simulink model "GFLI_L"  (R2024b)
settings: Solver=ode4  StartTime=0.0  StopTime=13  FixedStep=Tsam  RelTol=1e-3
values from neighbouring files (symbols this model uses):
  I2d = 3195    [GFLI_meas.m]    (also in SameOP_DifferParams.m; SameOP_Params_DifferConfig.m)
  I2q = -2132    [GFLI_meas.m]    (also in SameOP_DifferParams.m = 0; SameOP_Params_DifferConfig.m = 0)
  Kii = 0.0348    [GFLI_meas.m]
  Kipll = 400/(Vdc/2)    (= 0.695652173913)    [GFLI_meas.m]
  Kpi = 1.7391e-4    (= 0.00017391)    [GFLI_meas.m]
  Kppll = 40/(Vdc/2)    (= 0.0695652173913)    [GFLI_meas.m]
  Lf1 = 250e-6    (= 0.00025)    [GFLI_meas.m]
  Rf1 = 3e-3    (= 0.003)    [GFLI_meas.m]
  s = tf('s')    [GFLI_meas.m]    (also in GFLI_meas_PlotYddYqq.m; SameOP_DifferParams.m)
  Td = 1.5*Ts    (= 0.0003)    [GFLI_meas.m]    (also in GFLI_meas_PlotYddYqq.m = p.Td; SameOP_DifferParams.m = p.Td)
  Tsam = 5e-5    (= 5e-05)    [GFLI_meas.m]
  Vdc = 1150    [GFLI_meas.m]
  Vg = 575    [GFLI_meas.m]
  w = w_meas    [GFLI_meas.m]
  w1 = 2*pi*f0    (= 314.159265359)    [GFLI_meas.m]    (also in GFLI_meas_PlotYddYqq.m)
  w_meas = 2*pi*fHz_meas    [GFLI_meas.m]    (also in GFLI_meas_PlotYddYqq.m; SameOP_DifferParams.m; SameOP_Params_DifferConfig.m)
undefined symbols (not defined in the file or in its folder): DiscIntNeverNeededParam
libraries: slctrl_fre x12, spsControlledVoltageSourceLib x6, spsabctodq0Lib x5, slctrl_signal x4, spsACVoltageSourceLib x3, spsSeriesRLCBranchLib x3, spsdq0toabcLib x2, spsThreePhaseVIMeasurementLib x2, spsPLL3phLib x1, spsGroundLib x1, sps_lib x1
(part 1 of 2)
settings Model: SimulationMode=accelerator  Creator=ACER  LastModifiedBy=ACER
settings DataIOCC: SaveFormat=StructureWithTime  SignalLogging=off  DSMLogging=off  SaveTime=off  ReturnWorkspaceOutputs=off

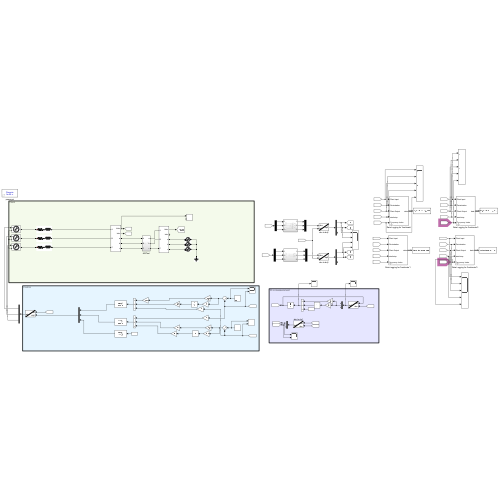
[thumbnail: Simulink's stored preview of the top-level diagram]
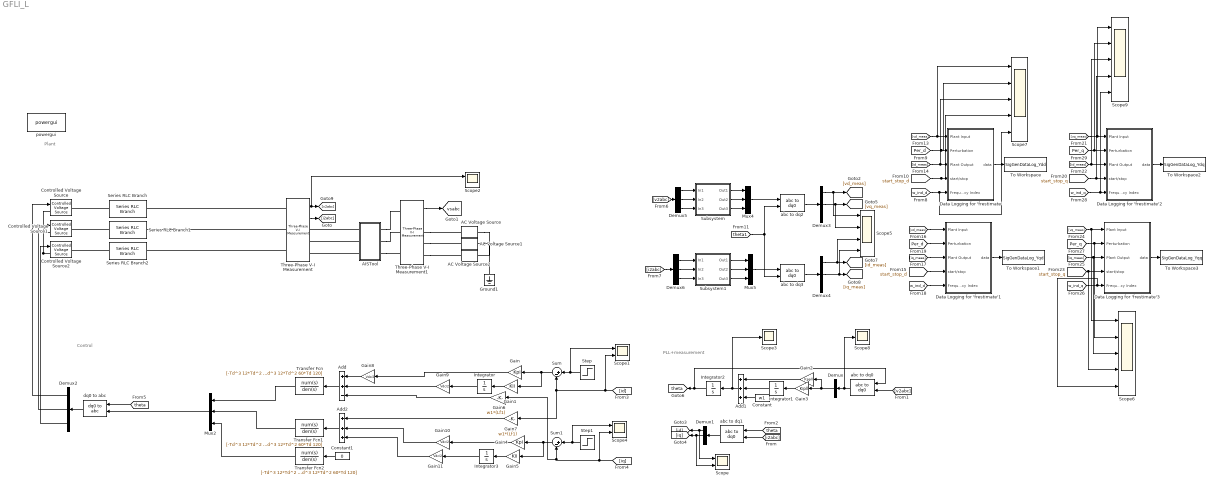
== system GFLI_L ==
  note: Plant
  note: Control
  note: PLL+measurement
  AC Voltage Source : spsACVoltageSourceLib/AC Voltage Source  Amplitude=Vg  Phase=0  Frequency=50  SampleTime=0  Measurements=None  BusType=swing  Pref=10e3  Qref=0  Qmin=-inf  Qmax=+inf
  AC Voltage Source1 : spsACVoltageSourceLib/AC Voltage Source  Amplitude=Vg  Phase=-120  Frequency=50  SampleTime=0  Measurements=None  BusType=swing  Pref=10e3  Qref=0  Qmin=-inf  Qmax=+inf
  AC Voltage Source2 : spsACVoltageSourceLib/AC Voltage Source  Amplitude=Vg  Phase=120  Frequency=50  SampleTime=0  Measurements=None  BusType=swing  Pref=10e3  Qref=0  Qmin=-inf  Qmax=+inf
  AISTool : Subsystem
  Add : Sum  Inputs=++-
  Add1 : Sum  Inputs=+++
  Add2 : Sum  Inputs=+++
  Constant : Constant  Value=w1
  Constant1 : Constant  Value=0
  Controlled Voltage Source : spsControlledVoltageSourceLib/Controlled Voltage Source  Initialize=on  Source_Type=AC  Amplitude=0  Phase=0  Frequency=0  Measurements=None
  Controlled Voltage Source1 : spsControlledVoltageSourceLib/Controlled Voltage Source  Initialize=on  Source_Type=AC  Amplitude=0  Phase=0  Frequency=0  Measurements=None
  Controlled Voltage Source2 : spsControlledVoltageSourceLib/Controlled Voltage Source  Initialize=on  Source_Type=AC  Amplitude=0  Phase=0  Frequency=0  Measurements=None
  Data Logging for 'frestimate' : Subsystem  mask(Companion Data Logger){Ts=Tsam, SignalType=Sinestream, FrequenciesSS=w_meas, FreqUnitsSS=rad/s, NumOfSetPeriod=1, NumOfEstPeriod=2, PRBSNumOfPeriod=1, FrequenciesSI=w, FreqUnitsSI=rad/s, NumOfPeriodLowestFreq=3, ReadySignalActiveChoice=VariantSinestream, InfoSignalActiveChoice=VariantSinestream}
      mask prompts: Ts "Sample Time (Ts)"; SignalType "Input Signal Type"; FrequenciesSS "Frequencies Vector"; NumOfSetPeriod "Number of Settling Periods"; NumOfEstPeriod "Number of Estimation Periods"; PRBSNumOfPeriod "Number of PRBS Signal Periods"; FrequenciesSI "Frequencies Vector"; NumOfPeriodLowestFreq "Number of  periods of the lowest frequency"; ReadySignalActiveChoice "Simulink:Variants:LabelComboBox"; InfoSignalActiveChoice "Simulink:Variants:LabelComboBox"
      mask help: Log data from signal generator blocks to work with "frestimate" API or frequency response estimation.
      mask init:
      | IsSinestreamSignal = strcmpi(get_param(gcb,'SignalType'),'Sinestream');
      |     IsSuperpositionSignal = strcmpi(get_param(gcb,'SignalType'),'Superposition');
      |     IsPRBSSignal = strcmpi(get_param(gcb,'SignalType'),'PRBS');
      |     IsHz = false;
      |     maskObj = Simulink.Mask.get(gcb);
      |     objectSinestream = maskObj.getDialogControl('SinestreamPanel');
      |     objectSuperposition = maskObj.getDialogControl('SuperpositionPanel');
      |     objectPRBS = maskObj.getDialogControl('PRBSPanel');
      |     %% Update optional inports
      |     inport_name = {'Frequency Index'};
      |     AvailableBlocks = get_param(gcb,'Blocks');
      |     % what exists in the block (old)
      |     type_in_block = ismember(inport_name,AvailableBlocks);
      |     % what is specified in the dialog (new)
      |     type_in_mask = IsSinestreamSignal;
      |     if IsSinestreamSignal
      |         objectSinestream.Visible = 'on';
      |         objectSuperposition.Visible = 'off';
      |         objectPRBS.Visible = 'off';
      |         set_param(gcb,'ReadySignalActiveChoice','VariantSinestream');  
      |         set_param(gcb,'InfoSignalActiveChoice','VariantSinestream');        
      |         IsHz = strcmpi(get_param(gcb,'FreqUnitsSS'),'Hz');
      |     elseif IsPRBSSignal
      |         objectSinestream.Visible = 'off';
      |         objectSuperposition.Visible = 'off';
      |         objectPRBS.Visible = 'on';
      |         set_param(gcb,'ReadySignalActiveChoice','VariantPRBS');  
      |         set_param(gcb,'InfoSignalActiveChoice','VariantPRBS');    
      |     else
      |         objectSinestream.Visible = 'off';
      |         objectSuperposition.Visible = 'on';
      |         objectPRBS.Visible = 'off';
      |         set_param(gcb,'ReadySignalActiveChoice','VariantSuperposition');  
      |         set_param(gcb,'InfoSignalActiveChoice','VariantSuperposition');    
      |         IsHz = strcmpi(get_param(gcb,'FreqUnitsSI'),'Hz');
      |     end
      |     % Update Inport
      |     port = 5;
      |     port = slctrlblkdlgs.OnlinePIDTuner.utilUpdateInport(gcb,'RateTransition_idx',AvailableBlocks,type_in_mask,type_in_block,1,'Frequency Index',port,1,'FrequenciesSS','double');
      |     if IsHz
      |         ConvFactor = 2*pi;
      |     else
      |         ConvFactor = 1;
      |     end
      mask Help: eval(open("block_data_logging_for_frestimate.html"));
      mask TypeOptions SignalType: Sinestream | Superposition | PRBS
      mask TypeOptions FreqUnitsSS: rad/s | Hz
      mask TypeOptions FreqUnitsSI: rad/s | Hz
      mask TypeOptions ReadySignalActiveChoice: Generate Ready Signal/LabelModeActiveChoice
      mask TypeOptions InfoSignalActiveChoice: Generate Info Signal/LabelModeActiveChoice
      mask DialogControl Container3 Prompt: Signal Specific Settings
      mask DialogControl ReadySignalActiveChoice Prompt: Label mode active choice:
      mask DialogControl InfoSignalActiveChoice Prompt: Label mode active choice:
  Data Logging for 'frestimate'1 : Subsystem  mask(Companion Data Logger){Ts=Tsam, SignalType=Sinestream, FrequenciesSS=w_meas, FreqUnitsSS=rad/s, NumOfSetPeriod=1, NumOfEstPeriod=2, PRBSNumOfPeriod=1, FrequenciesSI=w, FreqUnitsSI=rad/s, NumOfPeriodLowestFreq=3, ReadySignalActiveChoice=VariantSinestream, InfoSignalActiveChoice=VariantSinestream}
      mask prompts: Ts "Sample Time (Ts)"; SignalType "Input Signal Type"; FrequenciesSS "Frequencies Vector"; NumOfSetPeriod "Number of Settling Periods"; NumOfEstPeriod "Number of Estimation Periods"; PRBSNumOfPeriod "Number of PRBS Signal Periods"; FrequenciesSI "Frequencies Vector"; NumOfPeriodLowestFreq "Number of  periods of the lowest frequency"; ReadySignalActiveChoice "Simulink:Variants:LabelComboBox"; InfoSignalActiveChoice "Simulink:Variants:LabelComboBox"
      mask help: Log data from signal generator blocks to work with "frestimate" API or frequency response estimation.
      mask init: same as GFLI_L/Data Logging for 'frestimate'
      mask Help: eval(open("block_data_logging_for_frestimate.html"));
      mask TypeOptions SignalType: Sinestream | Superposition | PRBS
      mask TypeOptions FreqUnitsSS: rad/s | Hz
      mask TypeOptions FreqUnitsSI: rad/s | Hz
      mask TypeOptions ReadySignalActiveChoice: Generate Ready Signal/LabelModeActiveChoice
      mask TypeOptions InfoSignalActiveChoice: Generate Info Signal/LabelModeActiveChoice
      mask DialogControl Container3 Prompt: Signal Specific Settings
      mask DialogControl ReadySignalActiveChoice Prompt: Label mode active choice:
      mask DialogControl InfoSignalActiveChoice Prompt: Label mode active choice:
  Data Logging for 'frestimate'2 : Subsystem  mask(Companion Data Logger){Ts=Tsam, SignalType=Sinestream, FrequenciesSS=w_meas, FreqUnitsSS=rad/s, NumOfSetPeriod=1, NumOfEstPeriod=2, PRBSNumOfPeriod=1, FrequenciesSI=w, FreqUnitsSI=rad/s, NumOfPeriodLowestFreq=3, ReadySignalActiveChoice=VariantSinestream, InfoSignalActiveChoice=VariantSinestream}
      mask prompts: Ts "Sample Time (Ts)"; SignalType "Input Signal Type"; FrequenciesSS "Frequencies Vector"; NumOfSetPeriod "Number of Settling Periods"; NumOfEstPeriod "Number of Estimation Periods"; PRBSNumOfPeriod "Number of PRBS Signal Periods"; FrequenciesSI "Frequencies Vector"; NumOfPeriodLowestFreq "Number of  periods of the lowest frequency"; ReadySignalActiveChoice "Simulink:Variants:LabelComboBox"; InfoSignalActiveChoice "Simulink:Variants:LabelComboBox"
      mask help: Log data from signal generator blocks to work with "frestimate" API or frequency response estimation.
      mask init: same as GFLI_L/Data Logging for 'frestimate'
      mask Help: eval(open("block_data_logging_for_frestimate.html"));
      mask TypeOptions SignalType: Sinestream | Superposition | PRBS
      mask TypeOptions FreqUnitsSS: rad/s | Hz
      mask TypeOptions FreqUnitsSI: rad/s | Hz
      mask TypeOptions ReadySignalActiveChoice: Generate Ready Signal/LabelModeActiveChoice
      mask TypeOptions InfoSignalActiveChoice: Generate Info Signal/LabelModeActiveChoice
      mask DialogControl Container3 Prompt: Signal Specific Settings
      mask DialogControl ReadySignalActiveChoice Prompt: Label mode active choice:
      mask DialogControl InfoSignalActiveChoice Prompt: Label mode active choice:
  Data Logging for 'frestimate'3 : Subsystem  mask(Companion Data Logger){Ts=Tsam, SignalType=Sinestream, FrequenciesSS=w_meas, FreqUnitsSS=rad/s, NumOfSetPeriod=1, NumOfEstPeriod=2, PRBSNumOfPeriod=1, FrequenciesSI=w, FreqUnitsSI=rad/s, NumOfPeriodLowestFreq=3, ReadySignalActiveChoice=VariantSinestream, InfoSignalActiveChoice=VariantSinestream}
      mask prompts: Ts "Sample Time (Ts)"; SignalType "Input Signal Type"; FrequenciesSS "Frequencies Vector"; NumOfSetPeriod "Number of Settling Periods"; NumOfEstPeriod "Number of Estimation Periods"; PRBSNumOfPeriod "Number of PRBS Signal Periods"; FrequenciesSI "Frequencies Vector"; NumOfPeriodLowestFreq "Number of  periods of the lowest frequency"; ReadySignalActiveChoice "Simulink:Variants:LabelComboBox"; InfoSignalActiveChoice "Simulink:Variants:LabelComboBox"
      mask help: Log data from signal generator blocks to work with "frestimate" API or frequency response estimation.
      mask init: same as GFLI_L/Data Logging for 'frestimate'
      mask Help: eval(open("block_data_logging_for_frestimate.html"));
      mask TypeOptions SignalType: Sinestream | Superposition | PRBS
      mask TypeOptions FreqUnitsSS: rad/s | Hz
      mask TypeOptions FreqUnitsSI: rad/s | Hz
      mask TypeOptions ReadySignalActiveChoice: Generate Ready Signal/LabelModeActiveChoice
      mask TypeOptions InfoSignalActiveChoice: Generate Info Signal/LabelModeActiveChoice
      mask DialogControl Container3 Prompt: Signal Specific Settings
      mask DialogControl ReadySignalActiveChoice Prompt: Label mode active choice:
      mask DialogControl InfoSignalActiveChoice Prompt: Label mode active choice:
  Demux{,1..6} (7 alike) : Demux  Outputs=3
  Gain : Gain  Gain=Kpi
  Gain1 : Gain  Gain=Kii
  Gain{8..11} (4 alike) : Gain  Gain=Vdc/2
  Gain2 : Gain  Gain=Kppll
  Gain3 : Gain  Gain=Kipll
  Gain4 : Gain  Gain=Kpi
  Gain5 : Gain  Gain=Kii
  Gain6 : Gain  Gain=w1*(Lf1)
  Gain7 : Gain  Gain=w1*(Lf1)
  Ground1 : spsGroundLib/Ground  LConnTagsString=a
  Integrator{,1..3} (4 alike) : Integrator
  Mux2 : Mux  Inputs=3
  Mux4 : Mux  Inputs=3
  Mux5 : Mux  Inputs=3
  Scope{,1..2,4} (4 alike) : Scope  NumInputPorts=2
  Scope3 : Scope
  Scope5 : Scope  NumInputPorts=4
  Scope6 : Scope  NumInputPorts=5
  Scope7 : Scope  NumInputPorts=5
  Scope8 : Scope
  Scope9 : Scope  NumInputPorts=5
  Series RLC Branch : spsSeriesRLCBranchLib/Series RLC Branch  LConnTagsString=__new0  RConnTagsString=__new0  BranchType=RL  Resistance=Rf1  Inductance=Lf1  SetiL0=off  InitialCurrent=0  Capacitance=1e-6  Setx0=off  InitialVoltage=0  Measurements=None
  Series RLC Branch1 : spsSeriesRLCBranchLib/Series RLC Branch  LConnTagsString=__new0  RConnTagsString=__new0  BranchType=RL  Resistance=Rf1  Inductance=Lf1  SetiL0=off  InitialCurrent=0  Capacitance=1e-6  Setx0=off  InitialVoltage=0  Measurements=None
  Series RLC Branch2 : spsSeriesRLCBranchLib/Series RLC Branch  LConnTagsString=__new0  RConnTagsString=__new0  BranchType=RL  Resistance=Rf1  Inductance=Lf1  SetiL0=off  InitialCurrent=0  Capacitance=1e-6  Setx0=off  InitialVoltage=0  Measurements=None
  Step : Step  Time=2  Before=I2d  After=I2d  SampleTime=0
  Step1 : Step  Time=3  Before=I2q  After=I2q  SampleTime=0
  Subsystem : Subsystem
  Subsystem1 : Subsystem
  Sum : Sum  Inputs=|+-
  Sum1 : Sum  Inputs=|+-
  Three-Phase V-I Measurement : spsThreePhaseVIMeasurementLib/Three-Phase V-I Measurement  VoltageMeasurement=phase-to-ground  SetLabelV=off  LabelV=Vabc  Vpu=off  VpuLL=off  CurrentMeasurement=yes  SetLabelI=off  LabelI=Iabc  Ipu=off  Pbase=100e6  Vbase=500e3  OutputType=Complex  PhasorSimulation=off  PSBequivalent=0
  Three-Phase V-I Measurement1 : spsThreePhaseVIMeasurementLib/Three-Phase V-I Measurement  VoltageMeasurement=phase-to-ground  SetLabelV=off  LabelV=Vabc  Vpu=off  VpuLL=off  CurrentMeasurement=yes  SetLabelI=off  LabelI=Iabc  Ipu=off  Pbase=100e6  Vbase=500e3  OutputType=Complex  PhasorSimulation=off  PSBequivalent=0
  To Workspace : ToWorkspace  VariableName=SigGenDataLog_Ydd  SaveFormat=Timeseries  SampleTime=5e-5
  To Workspace1 : ToWorkspace  VariableName=SigGenDataLog_Yqd  SaveFormat=Timeseries  SampleTime=5e-5
  To Workspace2 : ToWorkspace  VariableName=SigGenDataLog_Ydq  SaveFormat=Timeseries  SampleTime=5e-5
  To Workspace3 : ToWorkspace  VariableName=SigGenDataLog_Yqq  SaveFormat=Timeseries  SampleTime=5e-5
  Transfer Fcn : TransferFcn  Numerator=[-Td^3 12*Td^2 -60*Td 120]  Denominator=[Td^3 12*Td^2 60*Td 120]
  Transfer Fcn1 : TransferFcn  Numerator=[-Td^3 12*Td^2 -60*Td 120]  Denominator=[Td^3 12*Td^2 60*Td 120]
  Transfer Fcn2 : TransferFcn  Numerator=[-Td^3 12*Td^2 -60*Td 120]  Denominator=[Td^3 12*Td^2 60*Td 120]
  abc to dq{0..3} (4 alike) : spsabctodq0Lib/abc to dq0  Alignment=Aligned with phase A axis
  dq0 to abc : spsdq0toabcLib/dq0 to abc  Alignment=Aligned with phase A axis
  powergui : sps_lib/powergui  Priority=1  SimulationMode=Discrete  SampleTime=Tsam  frequency=60  Iterations=50  frequencyindice=0  Pbase=100e6  ErrMax=1e-4  UnitsV=kV  UnitsW=MW  buscounter=0  FunctionMessages=off  echomessages=off  EnableUseOfTLC=off  CurrentSourceSwitches=off  DisableSnubberDevices=off  DisableRonSwitches=off  DisableVfSwitches=off  DisplayEquations=off  AutomaticDiscreteSolvers=off  SolverType=Tustin/Backward Euler (TBE)  Interpol=off  ExternalGateDelay=off  methode=off  Ts=100  x0status=zero  SPID=on  SwTol=0  HookPort=off  NonlinearTolerance=1e-4  nMaxIteration=100  ContinueOnMaxIteration=off  RestoreLinks=warning  ResistiveCurrentMeasurement=off  Frange=[0:2:500]  Ylog=off  Xlog=on  ShowGrid=off  save=off  variable=ZData  structure=0  ZoomFFT=off  StartTime=0.0  cycles=1  DisplayStyle=1  fundamental=60  FreqAxis=off  MaxFrequency=1000  frequencyindicesteady=1  RmsSteady=1  display=off
  tag scope: theta=global, vsabc=global
  wires:
  Demux1/2 -> Scope/2, [iq]
  Mux2/1 -> dq0 to abc/1
  Demux/2 -> Gain2/1, Gain3/1
  Demux2/3 -> Controlled Voltage Source2/1
  [theta] -> dq0 to abc/2
  Gain5/1 -> Integrator3/1
  Integrator2/1 -> [theta], abc to dq0/2
  dq0 to abc/1 -> Demux2/1
  Add2/1 -> Transfer Fcn1/1
  [theta] -> abc to dq1/2
  Demux2/2 -> Controlled Voltage Source1/1
  Gain/1 -> Gain8/1
  Add/1 -> Transfer Fcn/1
  Gain9/1 -> Add/2
  Integrator3/1 -> Gain11/1
  [iq] -> Scope4/2, Gain6/1, Sum1/2
  Add1/1 -> Scope3/1, Integrator2/1
  Transfer Fcn2/1 -> Mux2/3
  Gain1/1 -> Integrator/1
  Transfer Fcn/1 -> Mux2/1
  [i2abc] -> abc to dq1/1
  Sum1/1 -> Gain4/1, Gain5/1
  Gain8/1 -> Add/1
  Sum/1 -> Gain1/1, Gain/1
  Gain4/1 -> Gain10/1
  Gain11/1 -> Add2/3
  Constant/1 -> Add1/3
  Step1/1 -> Scope4/1, Sum1/1
  Integrator1/1 -> Add1/2
  Gain2/1 -> Add1/1
  Gain3/1 -> Integrator1/1
  abc to dq0/1 -> Scope8/1, Demux/1
  Transfer Fcn1/1 -> Mux2/2
  Demux1/1 -> Scope/1, [id]
  Constant1/1 -> Transfer Fcn2/1
  Demux2/1 -> Controlled Voltage Source/1
  Step/1 -> Scope1/1, Sum/1
  [id] -> Scope1/2, Gain7/1, Sum/2
  abc to dq1/1 -> Demux1/1
  Integrator/1 -> Gain9/1
  Gain10/1 -> Add2/2
  [v2abc] -> abc to dq0/1
  Data Logging for 'frestimate'/1(data) -> To Workspace/1
  abc to dq2/1 -> Demux3/1
  abc to dq3/1 -> Demux4/1
  Demux3/1 -> Scope5/1, [vd_meas]
  Demux3/2 -> Scope5/2, [vq_meas]
  Demux4/1 -> Scope5/3, [id_meas]
  Demux4/2 -> Scope5/4, [iq_meas]
  [w_ind_d] -> Scope7/5, Data Logging for 'frestimate'/5(Frequency Index)
  [Per_d] -> Scope7/2, Data Logging for 'frestimate'/2(Perturbation)
  [start_stop_d] -> Scope7/4, Data Logging for 'frestimate'/4(start/stop)
  [theta1] -> abc to dq3/2, abc to dq2/2
  [v2abc] -> Demux5/1
  Demux5/1 -> Subsystem/1(In1)
  Demux5/2 -> Subsystem/2(In2)
  Demux5/3 -> Subsystem/3(In3)
  Subsystem/2(Out2) -> Mux4/2
  Subsystem/1(Out1) -> Mux4/1
  Subsystem/3(Out3) -> Mux4/3
  Mux4/1 -> abc to dq2/1
  [i2abc] -> Demux6/1
  Demux6/2 -> Subsystem1/2(In2)
  Demux6/1 -> Subsystem1/1(In1)
  Demux6/3 -> Subsystem1/3(In3)
  Subsystem1/2(Out2) -> Mux5/2
  Subsystem1/1(Out1) -> Mux5/1
  Subsystem1/3(Out3) -> Mux5/3
  Mux5/1 -> abc to dq3/1
  [vd_meas] -> Scope7/1, Data Logging for 'frestimate'/1(Plant Input)
  [id_meas] -> Scope7/3, Data Logging for 'frestimate'/3(Plant Output)
  [iq_meas] -> Data Logging for 'frestimate'1/3(Plant Output)
  [vd_meas] -> Data Logging for 'frestimate'1/1(Plant Input)
  [start_stop_d] -> Data Logging for 'frestimate'1/4(start/stop)
  [Per_d] -> Data Logging for 'frestimate'1/2(Perturbation)
  [w_ind_d] -> Data Logging for 'frestimate'1/5(Frequency Index)
  Data Logging for 'frestimate'1/1(data) -> To Workspace1/1
  Data Logging for 'frestimate'3/1(data) -> To Workspace3/1
  [w_ind_q] -> Scope6/5, Data Logging for 'frestimate'3/5(Frequency Index)
  [Per_q] -> Data Logging for 'frestimate'3/2(Perturbation), Scope6/2
  [start_stop_q] -> Scope6/4, Data Logging for 'frestimate'3/4(start/stop)
  [vq_meas] -> Data Logging for 'frestimate'3/1(Plant Input), Scope6/1
  [iq_meas] -> Data Logging for 'frestimate'3/3(Plant Output), Scope6/3
  [id_meas] -> Scope9/3, Data Logging for 'frestimate'2/3(Plant Output)
  [vq_meas] -> Scope9/1, Data Logging for 'frestimate'2/1(Plant Input)
  [start_stop_q] -> Scope9/4, Data Logging for 'frestimate'2/4(start/stop)
  [Per_q] -> Scope9/2, Data Logging for 'frestimate'2/2(Perturbation)
  [w_ind_q] -> Scope9/5, Data Logging for 'frestimate'2/5(Frequency Index)
  Data Logging for 'frestimate'2/1(data) -> To Workspace2/1
  Three-Phase V-I Measurement/2 -> [i2abc]
  Three-Phase V-I Measurement/1 -> Scope2/1, [v2abc]
  Gain6/1 -> Add/3
  Gain7/1 -> Add2/1
  Three-Phase V-I Measurement1/1 -> [vsabc]
  connections:
  Controlled Voltage Source2/LConn1 -- Controlled Voltage Source/LConn1 -- Controlled Voltage Source1/LConn1
  Three-Phase V-I Measurement/LConn1 -- Series RLC Branch/RConn1
  AISTool/RConn1 -- Three-Phase V-I Measurement/RConn1
  Three-Phase V-I Measurement/LConn3 -- Series RLC Branch2/RConn1
  Series RLC Branch2/LConn1 -- Controlled Voltage Source2/RConn1
  Series RLC Branch1/RConn1 -- Three-Phase V-I Measurement/LConn2
  Series RLC Branch1/LConn1 -- Controlled Voltage Source1/RConn1
  Series RLC Branch/LConn1 -- Controlled Voltage Source/RConn1
  AISTool/RConn2 -- Three-Phase V-I Measurement/RConn2
  AISTool/RConn3 -- Three-Phase V-I Measurement/RConn3
  AC Voltage Source/LConn1 -- Ground1/LConn1 -- AC Voltage Source2/LConn1 -- AC Voltage Source1/LConn1
  AISTool/LConn2 -- Three-Phase V-I Measurement1/LConn2
  AISTool/LConn1 -- Three-Phase V-I Measurement1/LConn1
  AISTool/LConn3 -- Three-Phase V-I Measurement1/LConn3
  Three-Phase V-I Measurement1/RConn3 -- AC Voltage Source2/RConn1
  Three-Phase V-I Measurement1/RConn2 -- AC Voltage Source1/RConn1
  Three-Phase V-I Measurement1/RConn1 -- AC Voltage Source/RConn1

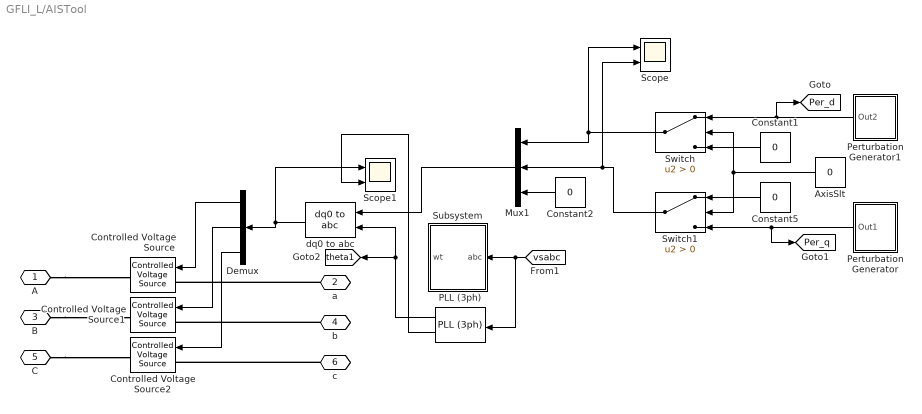
== system GFLI_L/AISTool ==
  AxisSlt : Constant  Value=0
  Constant1 : Constant  Value=0
  Constant2 : Constant  Value=0
  Constant5 : Constant  Value=0
  Controlled Voltage Source : spsControlledVoltageSourceLib/Controlled Voltage Source  Initialize=on  Source_Type=AC  Amplitude=0  Phase=0  Frequency=0  Measurements=None
  Controlled Voltage Source1 : spsControlledVoltageSourceLib/Controlled Voltage Source  Initialize=on  Source_Type=AC  Amplitude=0  Phase=0  Frequency=0  Measurements=None
  Controlled Voltage Source2 : spsControlledVoltageSourceLib/Controlled Voltage Source  Initialize=on  Source_Type=AC  Amplitude=0  Phase=0  Frequency=0  Measurements=None
  Demux : Demux  Outputs=3
  Mux1 : Mux  Inputs=3
  PLL (3ph) : spsPLL3phLib/PLL (3ph)  Fmin=45  Par_Init=[0, 50]  ParK=[180, 3200, 1]  TcD=1e-4  MaxRateChangeFreq=12  FilterCutOffFreq=25  Ts=0  AGC=on
      link override Model/Automatic Gain Control/Positive-Sequence (PLL-Driven)/abc ->dq0: Alignment=Aligned with phase A axis
      link override Model/abc to dq0: Alignment=Aligned with phase A axis
  Perturbation Generator : Subsystem
  Perturbation Generator1 : Subsystem
  Scope : Scope  NumInputPorts=2
  Scope1 : Scope  NumInputPorts=2
  Subsystem : Subsystem
  Switch : Switch  Criteria=u2 > Threshold  SaturateOnIntegerOverflow=off  InputSameDT=off
  Switch1 : Switch  Criteria=u2 > Threshold  SaturateOnIntegerOverflow=off  InputSameDT=off
  dq0 to abc : spsdq0toabcLib/dq0 to abc  Alignment=Aligned with phase A axis
  A : PMIOPort  Side=Right
  a : PMIOPort  Port=2  Side=Left
  B : PMIOPort  Port=3  Side=Right
  b : PMIOPort  Port=4  Side=Left
  C : PMIOPort  Port=5  Side=Right
  c : PMIOPort  Port=6  Side=Left
  tag scope: Per_d=global, Per_q=global, theta1=global
  wires:
  Demux/1 -> Controlled Voltage Source/1
  Demux/3 -> Controlled Voltage Source2/1
  Demux/2 -> Controlled Voltage Source1/1
  Constant1/1 -> Switch/3
  Constant5/1 -> Switch1/1
  AxisSlt/1 -> Switch/2, Switch1/2
  Perturbation Generator/1(Out1) -> [Per_q], Switch1/3
  Perturbation Generator1/1(Out2) -> [Per_d], Switch/1
  Mux1/1 -> dq0 to abc/1
  Constant2/1 -> Mux1/3
  Switch/1 -> Mux1/1, Scope/1
  Switch1/1 -> Scope/2, Mux1/2
  dq0 to abc/1 -> Demux/1, Scope1/1
  [vsabc] -> PLL (3ph)/1, Subsystem/1(abc)
  PLL (3ph)/1 -> Scope1/2
  PLL (3ph)/2 -> [theta1], dq0 to abc/2
  connections:
  b/RConn1 -- Controlled Voltage Source1/LConn1
  c/RConn1 -- Controlled Voltage Source2/LConn1
  B/RConn1 -- Controlled Voltage Source1/RConn1
  a/RConn1 -- Controlled Voltage Source/LConn1
  C/RConn1 -- Controlled Voltage Source2/RConn1
  A/RConn1 -- Controlled Voltage Source/RConn1

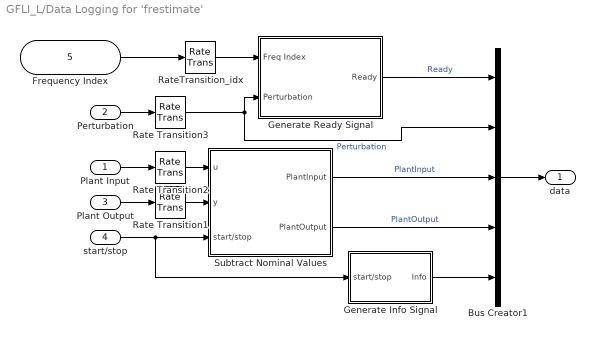
== system GFLI_L/Data Logging for 'frestimate' ==
  Plant Input : Inport
  Perturbation : Inport  Port=2
  Plant Output : Inport  Port=3
  start/stop : Inport  Port=4
  Frequency Index : Inport  Port=5
  Bus Creator1 : BusCreator  Inputs=5
  Generate Info Signal : Subsystem  Variant=on  VariantControlMode=label  LabelModeActiveChoice=VariantSinestream
  Generate Ready Signal : Subsystem  Variant=on  VariantControlMode=label  LabelModeActiveChoice=VariantSinestream
  Rate Transition1 : RateTransition  OutPortSampleTime=Ts
  Rate Transition2 : RateTransition  OutPortSampleTime=Ts
  Rate Transition3 : RateTransition  OutPortSampleTime=Ts
  RateTransition_idx : RateTransition  OutPortSampleTime=Ts
  Subtract Nominal Values : Subsystem
  data : Outport
  wires:
  Generate Info Signal/1(Info) -> Bus Creator1/5
  Bus Creator1/1 -> data/1
  Rate Transition3/1 -> Generate Ready Signal/2(Perturbation), Bus Creator1/2  "Perturbation"
  Subtract Nominal Values/1(PlantInput) -> Bus Creator1/3  "PlantInput"
  Subtract Nominal Values/2(PlantOutput) -> Bus Creator1/4  "PlantOutput"
  Generate Ready Signal/1(Ready) -> Bus Creator1/1  "Ready"
  Plant Output/1 -> Rate Transition1/1
  Plant Input/1 -> Rate Transition2/1
  start/stop/1 -> Generate Info Signal/1(start/stop), Subtract Nominal Values/3(start/stop)
  Rate Transition2/1 -> Subtract Nominal Values/1(u)
  Rate Transition1/1 -> Subtract Nominal Values/2(y)
  Perturbation/1 -> Rate Transition3/1
  RateTransition_idx/1 -> Generate Ready Signal/1(Freq Index)
  Frequency Index/1 -> RateTransition_idx/1

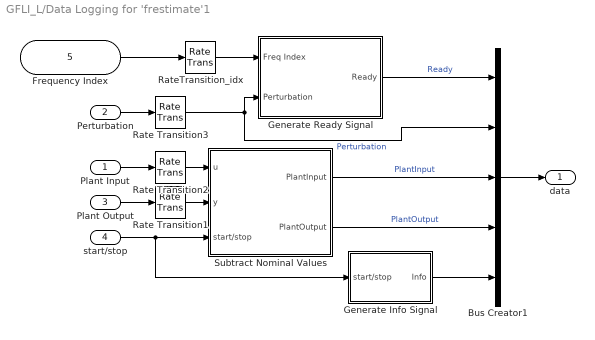
== system GFLI_L/Data Logging for 'frestimate'1 ==
  Plant Input : Inport
  Perturbation : Inport  Port=2
  Plant Output : Inport  Port=3
  start/stop : Inport  Port=4
  Frequency Index : Inport  Port=5
  Bus Creator1 : BusCreator  Inputs=5
  Generate Info Signal : Subsystem  Variant=on  VariantControlMode=label  LabelModeActiveChoice=VariantSinestream
  Generate Ready Signal : Subsystem  Variant=on  VariantControlMode=label  LabelModeActiveChoice=VariantSinestream
  Rate Transition1 : RateTransition  OutPortSampleTime=Ts
  Rate Transition2 : RateTransition  OutPortSampleTime=Ts
  Rate Transition3 : RateTransition  OutPortSampleTime=Ts
  RateTransition_idx : RateTransition  OutPortSampleTime=Ts
  Subtract Nominal Values : Subsystem
  data : Outport
  wires:
  Frequency Index/1 -> RateTransition_idx/1
  RateTransition_idx/1 -> Generate Ready Signal/1(Freq Index)
  Perturbation/1 -> Rate Transition3/1
  Rate Transition1/1 -> Subtract Nominal Values/2(y)
  Rate Transition2/1 -> Subtract Nominal Values/1(u)
  start/stop/1 -> Subtract Nominal Values/3(start/stop), Generate Info Signal/1(start/stop)
  Plant Input/1 -> Rate Transition2/1
  Plant Output/1 -> Rate Transition1/1
  Generate Ready Signal/1(Ready) -> Bus Creator1/1  "Ready"
  Subtract Nominal Values/2(PlantOutput) -> Bus Creator1/4  "PlantOutput"
  Subtract Nominal Values/1(PlantInput) -> Bus Creator1/3  "PlantInput"
  Rate Transition3/1 -> Bus Creator1/2, Generate Ready Signal/2(Perturbation)  "Perturbation"
  Bus Creator1/1 -> data/1
  Generate Info Signal/1(Info) -> Bus Creator1/5

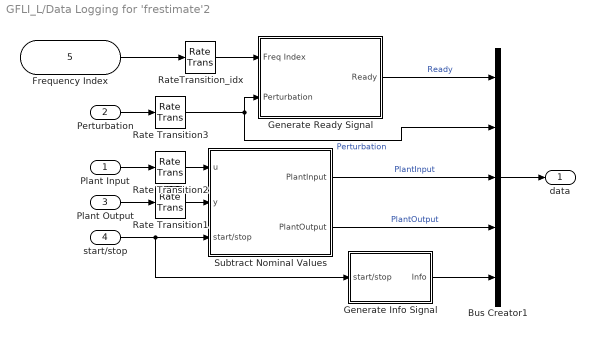
== system GFLI_L/Data Logging for 'frestimate'2 ==
  Plant Input : Inport
  Perturbation : Inport  Port=2
  Plant Output : Inport  Port=3
  start/stop : Inport  Port=4
  Frequency Index : Inport  Port=5
  Bus Creator1 : BusCreator  Inputs=5
  Generate Info Signal : Subsystem  Variant=on  VariantControlMode=label  LabelModeActiveChoice=VariantSinestream
  Generate Ready Signal : Subsystem  Variant=on  VariantControlMode=label  LabelModeActiveChoice=VariantSinestream
  Rate Transition1 : RateTransition  OutPortSampleTime=Ts
  Rate Transition2 : RateTransition  OutPortSampleTime=Ts
  Rate Transition3 : RateTransition  OutPortSampleTime=Ts
  RateTransition_idx : RateTransition  OutPortSampleTime=Ts
  Subtract Nominal Values : Subsystem
  data : Outport
  wires:
  Frequency Index/1 -> RateTransition_idx/1
  RateTransition_idx/1 -> Generate Ready Signal/1(Freq Index)
  Perturbation/1 -> Rate Transition3/1
  Rate Transition1/1 -> Subtract Nominal Values/2(y)
  Rate Transition2/1 -> Subtract Nominal Values/1(u)
  start/stop/1 -> Subtract Nominal Values/3(start/stop), Generate Info Signal/1(start/stop)
  Plant Input/1 -> Rate Transition2/1
  Plant Output/1 -> Rate Transition1/1
  Generate Ready Signal/1(Ready) -> Bus Creator1/1  "Ready"
  Subtract Nominal Values/2(PlantOutput) -> Bus Creator1/4  "PlantOutput"
  Subtract Nominal Values/1(PlantInput) -> Bus Creator1/3  "PlantInput"
  Rate Transition3/1 -> Bus Creator1/2, Generate Ready Signal/2(Perturbation)  "Perturbation"
  Bus Creator1/1 -> data/1
  Generate Info Signal/1(Info) -> Bus Creator1/5

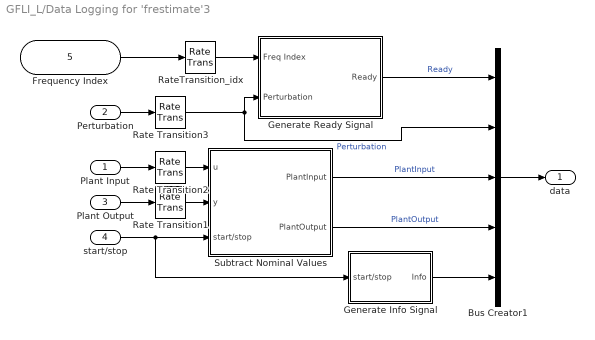
== system GFLI_L/Data Logging for 'frestimate'3 ==
  Plant Input : Inport
  Perturbation : Inport  Port=2
  Plant Output : Inport  Port=3
  start/stop : Inport  Port=4
  Frequency Index : Inport  Port=5
  Bus Creator1 : BusCreator  Inputs=5
  Generate Info Signal : Subsystem  Variant=on  VariantControlMode=label  LabelModeActiveChoice=VariantSinestream
  Generate Ready Signal : Subsystem  Variant=on  VariantControlMode=label  LabelModeActiveChoice=VariantSinestream
  Rate Transition1 : RateTransition  OutPortSampleTime=Ts
  Rate Transition2 : RateTransition  OutPortSampleTime=Ts
  Rate Transition3 : RateTransition  OutPortSampleTime=Ts
  RateTransition_idx : RateTransition  OutPortSampleTime=Ts
  Subtract Nominal Values : Subsystem
  data : Outport
  wires:
  Generate Info Signal/1(Info) -> Bus Creator1/5
  Bus Creator1/1 -> data/1
  Rate Transition3/1 -> Generate Ready Signal/2(Perturbation), Bus Creator1/2  "Perturbation"
  Subtract Nominal Values/1(PlantInput) -> Bus Creator1/3  "PlantInput"
  Subtract Nominal Values/2(PlantOutput) -> Bus Creator1/4  "PlantOutput"
  Generate Ready Signal/1(Ready) -> Bus Creator1/1  "Ready"
  Plant Output/1 -> Rate Transition1/1
  Plant Input/1 -> Rate Transition2/1
  start/stop/1 -> Generate Info Signal/1(start/stop), Subtract Nominal Values/3(start/stop)
  Rate Transition2/1 -> Subtract Nominal Values/1(u)
  Rate Transition1/1 -> Subtract Nominal Values/2(y)
  Perturbation/1 -> Rate Transition3/1
  RateTransition_idx/1 -> Generate Ready Signal/1(Freq Index)
  Frequency Index/1 -> RateTransition_idx/1

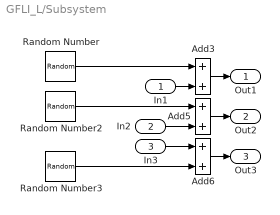
== system GFLI_L/Subsystem ==
  In1 : Inport
  In2 : Inport  Port=2
  In3 : Inport  Port=3
  Add3 : Sum
  Add5 : Sum
  Add6 : Sum
  Random Number : RandomNumber  Variance=(0.01*575)^2  Seed=23341  SampleTime=2e-4
  Random Number2 : RandomNumber  Variance=(0.01*575)^2  Seed=23342  SampleTime=2e-4
  Random Number3 : RandomNumber  Variance=(0.01*575)^2  Seed=23343  SampleTime=2e-4
  Out1 : Outport
  Out2 : Outport  Port=2
  Out3 : Outport  Port=3
  wires:
  In2/1 -> Add5/2
  Add5/1 -> Out2/1
  Add6/1 -> Out3/1
  Add3/1 -> Out1/1
  In1/1 -> Add3/2
  In3/1 -> Add6/1
  Random Number/1 -> Add3/1
  Random Number2/1 -> Add5/1
  Random Number3/1 -> Add6/2

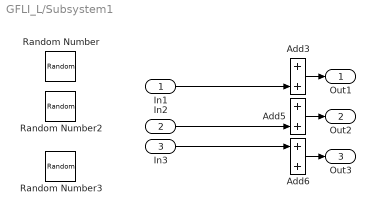
== system GFLI_L/Subsystem1 ==
  In1 : Inport
  In2 : Inport  Port=2
  In3 : Inport  Port=3
  Add3 : Sum
  Add5 : Sum
  Add6 : Sum
  Random Number : RandomNumber  Variance=(0.02*3195)^2  Seed=23341  SampleTime=2e-4
  Random Number2 : RandomNumber  Variance=(0.02*3195)^2  Seed=23342  SampleTime=2e-4
  Random Number3 : RandomNumber  Variance=(0.02*3195)^2  Seed=23343  SampleTime=2e-4
  Out1 : Outport
  Out2 : Outport  Port=2
  Out3 : Outport  Port=3
  wires:
  In3/1 -> Add6/1
  In1/1 -> Add3/2
  Add3/1 -> Out1/1
  Add6/1 -> Out3/1
  Add5/1 -> Out2/1
  In2/1 -> Add5/2

== system GFLI_L/AISTool/Perturbation Generator ==
  Constant1 : Constant
  Constant2 : Constant  Value=0.1
  Sinestream Signal Generator : slctrl_signal/Sinestream Signal Generator  DiscreteTs=Tsam  BlockDataType=double  SignalSource=Block parameters  Frequencies=w_meas  FreqUnits=rad/s  Amplitudes=28.75  NumOfFreq=3  NumOfSignalPeriod=3  SinestreamType=sine  PhaseShift=0  PhaseShiftUnits=deg  ThreePhaseSignal=off  OutputFreqIndex=on  UseExternalTs=off  CompiledTsChoice=InternalTs  SinestreamSignalChoice=VariantSin
      settings: LibrarySourceBlock=slctrlblks/Signal Generation/Sinestream Signal Generator
  Start-Stop Generator : slctrl_signal/Start-Stop Generator  DiscreteTs=Tsam  BlockDataType=double  StartStopTriggerMethod=External time vector  StartStopDuration=12.5  NumStartStopDelaySamples=2  SettlingTimeUpper=[1.1 2.1 3.1]  SettlingTimeLower=[0.9 1.9 2.9]  SettlingTimeInterval=5  StartStopTriggerSourceVariant=TimeBased
      settings: LibrarySourceBlock=slctrlblks/Signal Generation/Start-Stop Generator
  Out1 : Outport
  tag scope: start_stop_q=global, w_ind_q=global
  wires:
  Sinestream Signal Generator/1 -> Out1/1  "Current"
  Constant1/1 -> Start-Stop Generator/1
  Constant2/1 -> Start-Stop Generator/2
  Start-Stop Generator/1 -> [start_stop_q], Sinestream Signal Generator/1
  Sinestream Signal Generator/2 -> [w_ind_q]

== system GFLI_L/AISTool/Perturbation Generator1 ==
  Constant1 : Constant
  Constant2 : Constant  Value=0.1
  Sinestream Signal Generator : slctrl_signal/Sinestream Signal Generator  DiscreteTs=Tsam  BlockDataType=double  SignalSource=Block parameters  Frequencies=w_meas  FreqUnits=rad/s  Amplitudes=28.75  NumOfFreq=3  NumOfSignalPeriod=3  SinestreamType=sine  PhaseShift=0  PhaseShiftUnits=deg  ThreePhaseSignal=off  OutputFreqIndex=on  UseExternalTs=off  CompiledTsChoice=InternalTs  SinestreamSignalChoice=VariantSin
      settings: LibrarySourceBlock=slctrlblks/Signal Generation/Sinestream Signal Generator
  Start-Stop Generator : slctrl_signal/Start-Stop Generator  DiscreteTs=Tsam  BlockDataType=double  StartStopTriggerMethod=External time vector  StartStopDuration=12.5  NumStartStopDelaySamples=2  SettlingTimeUpper=[1.1 2.1 3.1]  SettlingTimeLower=[0.9 1.9 2.9]  SettlingTimeInterval=5  StartStopTriggerSourceVariant=TimeBased
      settings: LibrarySourceBlock=slctrlblks/Signal Generation/Start-Stop Generator
  Out2 : Outport
  tag scope: start_stop_d=global, w_ind_d=global
  wires:
  Sinestream Signal Generator/1 -> Out2/1  "Current"
  Sinestream Signal Generator/2 -> [w_ind_d]
  Constant2/1 -> Start-Stop Generator/2
  Constant1/1 -> Start-Stop Generator/1
  Start-Stop Generator/1 -> [start_stop_d], Sinestream Signal Generator/1

== system GFLI_L/AISTool/Subsystem ==
  abc : Inport
  Add1 : Sum  Inputs=+++
  Constant : Constant  Value=w1
  Demux1 : Demux  Outputs=3
  Gain2 : Gain  Gain=Kppll
  Gain3 : Gain  Gain=Kipll
  Integrator1 : Integrator
  Integrator2 : Integrator
  abc to dq0 : spsabctodq0Lib/abc to dq0  Alignment=Aligned with phase A axis
  wt : Outport
  wires:
  Gain2/1 -> Add1/1
  Gain3/1 -> Integrator1/1
  abc to dq0/1 -> Demux1/1
  Integrator1/1 -> Add1/2
  Constant/1 -> Add1/3
  Demux1/2 -> Gain2/1, Gain3/1
  Integrator2/1 -> wt/1, abc to dq0/2
  Add1/1 -> Integrator2/1
  abc/1 -> abc to dq0/1

== system GFLI_L/Data Logging for 'frestimate'/Generate Info Signal ==
  note: 1) Add Subsystem or Model blocks as valid variant choices.
      | 2) You cannot connect blocks at this level. At simulation, connectivity is automatically
      | determined, based on the active variant and port name matching.
  start/stop : Inport
  PRBS : Subsystem  VariantControl=VariantPRBS
  Sinestream : Subsystem  VariantControl=VariantSinestream
  Superposition : Subsystem  VariantControl=VariantSuperposition
  Info : Outport

== system GFLI_L/Data Logging for 'frestimate'/Generate Ready Signal ==
  note: 1) Add Subsystem or Model blocks as valid variant choices.
      | 2) You cannot connect blocks at this level. At simulation, connectivity is automatically
      | determined, based on the active variant and port name matching.
  Freq Index : Inport
  Perturbation : Inport  Port=2
  PRBS : Subsystem  VariantControl=VariantPRBS
  Sinestream : Subsystem  VariantControl=VariantSinestream
  Superposition : Subsystem  VariantControl=VariantSuperposition
  Ready : Outport

== system GFLI_L/Data Logging for 'frestimate'/Subtract Nominal Values ==
  u : Inport
  y : Inport  Port=2
  start/stop : Inport  Port=3
  Enabled Subsystem : Subsystem  TreatAsAtomicUnit=on
  PlantInput : Outport
  PlantOutput : Outport  Port=2
  wires:
  u/1 -> Enabled Subsystem/1(u)
  y/1 -> Enabled Subsystem/2(y)
  start/stop/1 -> Enabled Subsystem/3(start/stop), Enabled Subsystem/Enable
  Enabled Subsystem/1(PlantInput) -> PlantInput/1
  Enabled Subsystem/2(PlantOutput) -> PlantOutput/1

== system GFLI_L/Data Logging for 'frestimate'1/Generate Info Signal ==
  note: 1) Add Subsystem or Model blocks as valid variant choices.
      | 2) You cannot connect blocks at this level. At simulation, connectivity is automatically
      | determined, based on the active variant and port name matching.
  start/stop : Inport
  PRBS : Subsystem  VariantControl=VariantPRBS
  Sinestream : Subsystem  VariantControl=VariantSinestream
  Superposition : Subsystem  VariantControl=VariantSuperposition
  Info : Outport

== system GFLI_L/Data Logging for 'frestimate'1/Generate Ready Signal ==
  note: 1) Add Subsystem or Model blocks as valid variant choices.
      | 2) You cannot connect blocks at this level. At simulation, connectivity is automatically
      | determined, based on the active variant and port name matching.
  Freq Index : Inport
  Perturbation : Inport  Port=2
  PRBS : Subsystem  VariantControl=VariantPRBS
  Sinestream : Subsystem  VariantControl=VariantSinestream
  Superposition : Subsystem  VariantControl=VariantSuperposition
  Ready : Outport

== system GFLI_L/Data Logging for 'frestimate'1/Subtract Nominal Values ==
  u : Inport
  y : Inport  Port=2
  start/stop : Inport  Port=3
  Enabled Subsystem : Subsystem  TreatAsAtomicUnit=on
  PlantInput : Outport
  PlantOutput : Outport  Port=2
  wires:
  Enabled Subsystem/2(PlantOutput) -> PlantOutput/1
  Enabled Subsystem/1(PlantInput) -> PlantInput/1
  start/stop/1 -> Enabled Subsystem/Enable, Enabled Subsystem/3(start/stop)
  y/1 -> Enabled Subsystem/2(y)
  u/1 -> Enabled Subsystem/1(u)

== system GFLI_L/Data Logging for 'frestimate'2/Generate Info Signal ==
  note: 1) Add Subsystem or Model blocks as valid variant choices.
      | 2) You cannot connect blocks at this level. At simulation, connectivity is automatically
      | determined, based on the active variant and port name matching.
  start/stop : Inport
  PRBS : Subsystem  VariantControl=VariantPRBS
  Sinestream : Subsystem  VariantControl=VariantSinestream
  Superposition : Subsystem  VariantControl=VariantSuperposition
  Info : Outport

== system GFLI_L/Data Logging for 'frestimate'2/Generate Ready Signal ==
  note: 1) Add Subsystem or Model blocks as valid variant choices.
      | 2) You cannot connect blocks at this level. At simulation, connectivity is automatically
      | determined, based on the active variant and port name matching.
  Freq Index : Inport
  Perturbation : Inport  Port=2
  PRBS : Subsystem  VariantControl=VariantPRBS
  Sinestream : Subsystem  VariantControl=VariantSinestream
  Superposition : Subsystem  VariantControl=VariantSuperposition
  Ready : Outport

== system GFLI_L/Data Logging for 'frestimate'2/Subtract Nominal Values ==
  u : Inport
  y : Inport  Port=2
  start/stop : Inport  Port=3
  Enabled Subsystem : Subsystem  TreatAsAtomicUnit=on
  PlantInput : Outport
  PlantOutput : Outport  Port=2
  wires:
  Enabled Subsystem/2(PlantOutput) -> PlantOutput/1
  Enabled Subsystem/1(PlantInput) -> PlantInput/1
  start/stop/1 -> Enabled Subsystem/Enable, Enabled Subsystem/3(start/stop)
  y/1 -> Enabled Subsystem/2(y)
  u/1 -> Enabled Subsystem/1(u)

== system GFLI_L/Data Logging for 'frestimate'3/Generate Info Signal ==
  note: 1) Add Subsystem or Model blocks as valid variant choices.
      | 2) You cannot connect blocks at this level. At simulation, connectivity is automatically
      | determined, based on the active variant and port name matching.
  start/stop : Inport
  PRBS : Subsystem  VariantControl=VariantPRBS
  Sinestream : Subsystem  VariantControl=VariantSinestream
  Superposition : Subsystem  VariantControl=VariantSuperposition
  Info : Outport

== system GFLI_L/Data Logging for 'frestimate'3/Generate Ready Signal ==
  note: 1) Add Subsystem or Model blocks as valid variant choices.
      | 2) You cannot connect blocks at this level. At simulation, connectivity is automatically
      | determined, based on the active variant and port name matching.
  Freq Index : Inport
  Perturbation : Inport  Port=2
  PRBS : Subsystem  VariantControl=VariantPRBS
  Sinestream : Subsystem  VariantControl=VariantSinestream
  Superposition : Subsystem  VariantControl=VariantSuperposition
  Ready : Outport

== system GFLI_L/Data Logging for 'frestimate'3/Subtract Nominal Values ==
  u : Inport
  y : Inport  Port=2
  start/stop : Inport  Port=3
  Enabled Subsystem : Subsystem  TreatAsAtomicUnit=on
  PlantInput : Outport
  PlantOutput : Outport  Port=2
  wires:
  u/1 -> Enabled Subsystem/1(u)
  y/1 -> Enabled Subsystem/2(y)
  start/stop/1 -> Enabled Subsystem/3(start/stop), Enabled Subsystem/Enable
  Enabled Subsystem/1(PlantInput) -> PlantInput/1
  Enabled Subsystem/2(PlantOutput) -> PlantOutput/1

== system GFLI_L/Data Logging for 'frestimate'/Generate Info Signal/PRBS ==
  start/stop : Inport
  Info Bus : BusCreator  Inputs=1
  Info Snapshot : slctrl_fre/Frequency Response Estimator/Frequency Response Estimator/Variant Subsystem/PRBSNoEst/Info Snapshot  SystemSampleTime=-1  VariantActivationTime=update diagram  AllowFlexibleInterface=on  Latency=0  AutoFrameSizeCalculation=off
  PRBSNumPeriods : Constant  Value=PRBSNumOfPeriod  SampleTime=Ts
  Info : Outport
  wires:
  start/stop/1 -> Info Snapshot/Enable
  Info Snapshot/1 -> Info Bus/1  "PRBSNumPeriods"
  Info Bus/1 -> Info/1  "Info"
  PRBSNumPeriods/1 -> Info Snapshot/1

== system GFLI_L/Data Logging for 'frestimate'/Generate Info Signal/Sinestream ==
  start/stop : Inport
  Info Bus : BusCreator  Inputs=1
  Info Snapshot : slctrl_fre/Frequency Response Estimator/Frequency Response Estimator/Variant Subsystem/PRBSNoEst/Info Snapshot  SystemSampleTime=-1  VariantActivationTime=update diagram  AllowFlexibleInterface=on  Latency=0  AutoFrameSizeCalculation=off
  conversion factor : Gain  Gain=ConvFactor
  frequencies : Constant  Value=FrequenciesSS  SampleTime=Ts
  Info : Outport
  wires:
  Info Bus/1 -> Info/1  "Info"
  start/stop/1 -> Info Snapshot/Enable
  frequencies/1 -> conversion factor/1
  Info Snapshot/1 -> Info Bus/1  "frequencies"
  conversion factor/1 -> Info Snapshot/1

== system GFLI_L/Data Logging for 'frestimate'/Generate Info Signal/Superposition ==
  start/stop : Inport
  Info Bus : BusCreator  Inputs=1
  Info Snapshot : slctrl_fre/Frequency Response Estimator/Frequency Response Estimator/Variant Subsystem/PRBSNoEst/Info Snapshot  SystemSampleTime=-1  VariantActivationTime=update diagram  AllowFlexibleInterface=on  Latency=0  AutoFrameSizeCalculation=off
  conversion factor : Gain  Gain=ConvFactor
  frequencies : Constant  Value=FrequenciesSI  SampleTime=Ts
  Info : Outport
  wires:
  Info Snapshot/1 -> Info Bus/1  "frequencies"
  frequencies/1 -> conversion factor/1
  start/stop/1 -> Info Snapshot/Enable
  Info Bus/1 -> Info/1  "Info"
  conversion factor/1 -> Info Snapshot/1

== system GFLI_L/Data Logging for 'frestimate'/Generate Ready Signal/PRBS ==
  Freq Index : Inport
  Perturbation : Inport  Port=2
  Constant : Constant  Value=0  SampleTime=Ts
  Relational Operator : RelationalOperator  Operator=~=  OutDataTypeStr=boolean  RndMeth=Simplest  InputSameDT=off
  Terminator : Terminator
  Ready : Outport
  wires:
  Freq Index/1 -> Terminator/1
  Perturbation/1 -> Relational Operator/1  "Perturbation"
  Constant/1 -> Relational Operator/2
  Relational Operator/1 -> Ready/1  "Ready"

== system GFLI_L/Data Logging for 'frestimate'/Generate Ready Signal/Sinestream ==
  Freq Index : Inport
  Perturbation : Inport  Port=2
  ExtractReadySignal : Subsystem  mask(Extract Ready Signal){Ts=Ts, Frequencies=FrequenciesSS, NumOfSetPeriod=NumOfSetPeriod, NumOfEstPeriod=NumOfEstPeriod}
      mask prompts: Ts "Sample Time (Ts)"; Frequencies "Frequencies Vector"; NumOfSetPeriod "Number of Settling Periods"; NumOfEstPeriod "Number of Estimation Periods"
      mask help: Extract ready signal for the Sinestream Signal Generator block for offline frequency response estimation.
      mask init:
      | nw = length(Frequencies);
  Terminator : Terminator
  Ready : Outport
  wires:
  ExtractReadySignal/1(Ready Signal) -> Ready/1  "Ready"
  Perturbation/1 -> Terminator/1
  Freq Index/1 -> ExtractReadySignal/1(Frequency Index)

== system GFLI_L/Data Logging for 'frestimate'/Generate Ready Signal/Superposition ==
  Freq Index : Inport
  Perturbation : Inport  Port=2
  Constant : Constant  Value=0  SampleTime=Ts
  Relational Operator : RelationalOperator  Operator=~=  OutDataTypeStr=boolean  RndMeth=Simplest  InputSameDT=off
  Terminator : Terminator
  Ready : Outport
  wires:
  Relational Operator/1 -> Ready/1  "Ready"
  Constant/1 -> Relational Operator/2
  Perturbation/1 -> Relational Operator/1  "Perturbation"
  Freq Index/1 -> Terminator/1

== system GFLI_L/Data Logging for 'frestimate'/Subtract Nominal Values/Enabled Subsystem ==
  u : Inport
  y : Inport  Port=2
  start/stop : Inport  Port=3
  Enable : EnablePort
  ExtractNominalValues : Subsystem  mask(Remove Nominal Signal){Ts=Ts}
      mask prompts: Ts "Samplt Time (sec)"
      mask help: Remove nominal baseline signal from logged data.
  Sum : Sum  Inputs=|+-
  Sum1 : Sum  Inputs=-+|
  PlantInput : Outport
  PlantOutput : Outport  Port=2
  wires:
  start/stop/1 -> ExtractNominalValues/3(start/stop)
  Sum/1 -> PlantInput/1
  ExtractNominalValues/1(uNominal) -> Sum/2
  u/1 -> Sum/1, ExtractNominalValues/1(u)
  ExtractNominalValues/2(yNominal) -> Sum1/1
  y/1 -> Sum1/2, ExtractNominalValues/2(y)
  Sum1/1 -> PlantOutput/1

== system GFLI_L/Data Logging for 'frestimate'1/Generate Info Signal/PRBS ==
  start/stop : Inport
  Info Bus : BusCreator  Inputs=1
  Info Snapshot : slctrl_fre/Frequency Response Estimator/Frequency Response Estimator/Variant Subsystem/PRBSNoEst/Info Snapshot  SystemSampleTime=-1  VariantActivationTime=update diagram  AllowFlexibleInterface=on  Latency=0  AutoFrameSizeCalculation=off
  PRBSNumPeriods : Constant  Value=PRBSNumOfPeriod  SampleTime=Ts
  Info : Outport
  wires:
  PRBSNumPeriods/1 -> Info Snapshot/1
  Info Bus/1 -> Info/1  "Info"
  Info Snapshot/1 -> Info Bus/1  "PRBSNumPeriods"
  start/stop/1 -> Info Snapshot/Enable
